simulink library "carnotUIBK"  (R2024b)
settings: Solver=VariableStepAuto  StartTime=0.0  StopTime=10.0  RelTol=1e-3  EnableMultiTasking=on
values from neighbouring files (symbols this model uses):
  area = area + room(kk).area    [THERMALZONE.m]
  boundary = BOUNDARY()    [BUILDING.m]
  building = obj    [BUILDING.m]
  C = zeros(1,length(d)+1)    [CONSTRUCTION.m]
  cp = str2num(value)    [CONSTRUCTION.m]
  pos = find(d_layer>0)    [CONSTRUCTION.m]
  rho = str2num(value)    [CONSTRUCTION.m]
  type = 1    [CONSTRUCTION.m]
  zone = obj.zone(ind)    [THERMALZONE.m]
undefined symbols (not defined in the file or in its folder): A, amb_factor, B, const, control, Dd, get_building, height, p, Qdot_C, Qdot_H, Qdot_I_electricity, Qdot_I_light, Qdot_I_person, Qdot_S, Qdot_T_ground, Qdot_T_neighbour, Qdot_T_opaque, Qdot_T_window, Qdot_V_infiltration, Qdot_V_mech, Qdot_V_window, r_frame, solar_ratio, solar_ratio1, solar_ratio2, Tc, Tr, Ts, Uvalue, view_factor, wall, wallsurface, window, window_height, window_heigth, window_width, windowsurface, x_CO2, x_H2O, x_VOC, z
libraries: carnot x105, $bdroot x22, simulink x18, simulink_extras x14
(part 7 of 13)

== system carnotUIBK/gain/Light/W//light ==
  Switch : Inport
  Constant1 : Constant  Value=zeros(1,13)
  Constant2 : Constant  Value=zeros(1,3)
  Gain1 : Gain  Gain=0.6  SaturateOnIntegerOverflow=on  OutDataTypeStr=Inherit: Same as input  ParamDataTypeStr=Inherit: Same as input
  Gain4 : Gain  Gain=0.4  SaturateOnIntegerOverflow=on  OutDataTypeStr=Inherit: Same as input  ParamDataTypeStr=Inherit: Same as input
  Mux1 : Mux  Inputs=[1 1 13 1 3]
  Product1 : Product
  Profile W/light : carnot/Load/General/Repeating_Profile  period=timevalues(end)  rep_seq_t=timevalues(1:end-1)  rep_seq_d=timeduration  rep_seq_y=values1
      settings: SourceProductName=Carnot
  timeconstant : simulink_extras/Additional Linear/Transfer Fcn (with initial outputs)  N=[1]  D=[60 1]  Y0=0  U0=0
  "[S]" : Outport  VectorParamsAs1DForOutWhenUnconnected=off
  wires:
  Product1/1 -> "[S]"/1
  Switch/1 -> Product1/1
  Gain4/1 -> Mux1/2
  Mux1/1 -> Product1/2
  Gain1/1 -> Mux1/1
  Profile W/light/1 -> timeconstant/1
  Constant1/1 -> Mux1/3
  Constant2/1 -> Mux1/5
  timeconstant/1 -> Mux1/4, Gain4/1, Gain1/1

== system carnotUIBK/gain/Light/W//m² ==
  Switch : Inport
  Constant1 : Constant  Value=zeros(1,13)
  Constant2 : Constant  Value=zeros(1,3)
  Gain1 : Gain  Gain=z.heated_area  SaturateOnIntegerOverflow=on  OutDataTypeStr=Inherit: Same as input  ParamDataTypeStr=Inherit: Same as input
  Gain3 : Gain  Gain=0.6  SaturateOnIntegerOverflow=on  OutDataTypeStr=Inherit: Same as input  ParamDataTypeStr=Inherit: Same as input
  Gain5 : Gain  Gain=0.4  SaturateOnIntegerOverflow=on  OutDataTypeStr=Inherit: Same as input  ParamDataTypeStr=Inherit: Same as input
  Mux2 : Mux  Inputs=[1 1 13 1 3]
  Product : Product
  Profile W/m² : carnot/Load/General/Repeating_Profile  period=timevalues(end)  rep_seq_t=timevalues(1:end-1)  rep_seq_d=timeduration  rep_seq_y=values1
      settings: SourceProductName=Carnot
  timeconstant : simulink_extras/Additional Linear/Transfer Fcn (with initial outputs)  N=[1]  D=[60 1]  Y0=0  U0=0
  "[S]" : Outport  VectorParamsAs1DForOutWhenUnconnected=off
  wires:
  Product/1 -> "[S]"/1
  Switch/1 -> Product/1
  Gain5/1 -> Mux2/2
  Mux2/1 -> Product/2
  Gain3/1 -> Mux2/1
  Profile W/m²/1 -> Gain1/1
  Gain1/1 -> timeconstant/1
  Constant1/1 -> Mux2/3
  Constant2/1 -> Mux2/5
  timeconstant/1 -> Mux2/4, Gain5/1, Gain3/1

== system carnotUIBK/gain/Moisture/kg//s ==
  note: 2500 kJ/kg
  Constant13 : Constant  Value=zeros(1,11)
  Constant14 : Constant  Value=zeros(1,2)
  Constant3 : Constant  Value=zeros(1,2)
  Gain1 : Gain  Gain=1.0  SaturateOnIntegerOverflow=on  OutDataTypeStr=Inherit: Same as input  ParamDataTypeStr=Inherit: Same as input
  Gain2 : Gain  Gain=-2500000  SaturateOnIntegerOverflow=on  OutDataTypeStr=Inherit: Same as input  ParamDataTypeStr=Inherit: Same as input
  Gain4 : Gain  Gain=0.0  SaturateOnIntegerOverflow=on  OutDataTypeStr=Inherit: Same as input  ParamDataTypeStr=Inherit: Same as input
  Mux2 : Mux  Inputs=[1 1 2 1 11 1 2]
  Profile kg/s : carnot/Load/General/Repeating_Profile  period=timevalues(end)  rep_seq_t=timevalues(1:end-1)  rep_seq_d=timeduration  rep_seq_y=values1
      settings: SourceProductName=Carnot
  timeconstant : simulink_extras/Additional Linear/Transfer Fcn (with initial outputs)  N=[1]  D=[60 1]  Y0=0  U0=0
  "[S]" : Outport  VectorParamsAs1DForOutWhenUnconnected=off
  wires:
  Gain4/1 -> Mux2/2
  Mux2/1 -> "[S]"/1
  Gain1/1 -> Mux2/1
  Profile kg/s/1 -> timeconstant/1
  Constant13/1 -> Mux2/5
  Constant14/1 -> Mux2/7
  Constant3/1 -> Mux2/3
  Gain2/1 -> Mux2/6, Gain4/1, Gain1/1
  timeconstant/1 -> Mux2/4, Gain2/1

== system carnotUIBK/gain/People/W//m² ==
  Switch : Inport
  Constant1 : Constant  Value=zeros(1,12)
  Constant2 : Constant  Value=zeros(1,4)
  Gain1 : Gain  Gain=z.heated_area  SaturateOnIntegerOverflow=on  OutDataTypeStr=Inherit: Same as input  ParamDataTypeStr=Inherit: Same as input
  Gain2 : Gain  Gain=0.5  SaturateOnIntegerOverflow=on  OutDataTypeStr=Inherit: Same as input  ParamDataTypeStr=Inherit: Same as input
  Gain4 : Gain  Gain=0.5  SaturateOnIntegerOverflow=on  OutDataTypeStr=Inherit: Same as input  ParamDataTypeStr=Inherit: Same as input
  Mux1 : Mux  Inputs=[1 1 12 1 4]
  Product1 : Product
  profile_1 : carnot/Load/General/Repeating_Profile  period=timevalues(end)  rep_seq_t=timevalues(1:end-1)  rep_seq_d=timeduration  rep_seq_y=values1
      settings: SourceProductName=Carnot
  timeconstant : simulink_extras/Additional Linear/Transfer Fcn (with initial outputs)  N=[1]  D=[60 1]  Y0=0  U0=0
  "[S]" : Outport  VectorParamsAs1DForOutWhenUnconnected=off
  wires:
  Switch/1 -> Product1/1
  Product1/1 -> "[S]"/1
  Gain1/1 -> timeconstant/1
  Gain4/1 -> Mux1/2
  Gain2/1 -> Mux1/1
  Mux1/1 -> Product1/2
  profile_1/1 -> Gain1/1
  Constant1/1 -> Mux1/3
  Constant2/1 -> Mux1/5
  timeconstant/1 -> Gain4/1, Mux1/4, Gain2/1

== system carnotUIBK/gain/People/W//ppl (activity) ==
  Top : Inport
  Switch : Inport  Port=2
  Constant1 : Constant  Value=zeros(1,2)
  Constant2 : Constant  Value=zeros(1,4)
  Constant3 : Constant  Value=zeros(1,8)
  Gain1 : Gain  Gain=0.5  SaturateOnIntegerOverflow=on  OutDataTypeStr=Inherit: Same as input  ParamDataTypeStr=Inherit: Same as input
  Gain2 : Gain  Gain=0.5  SaturateOnIntegerOverflow=on  OutDataTypeStr=Inherit: Same as input  ParamDataTypeStr=Inherit: Same as input
  Gain4 : Gain  Gain=0.5  SaturateOnIntegerOverflow=on  OutDataTypeStr=Inherit: Same as input  ParamDataTypeStr=Inherit: Same as input
  LUT_Qdot_dry : Subsystem
      mask help:
      | This block delivers the SENSITIVE/DRY HEAT POWER one person emitts in a room depending on his activity and the actual sensitive temperature in the middle of a room.
      |
      | Qdot_dry	: sensitive/dry heat power emitted from 1 person, W
      | activity		: number of class of person activity (DIN 1946, VDI 2078):
      | 		   0 - no physical work (sleeping)
      | 		   1 - relaxed work (home, office, school)
      | 		   2 - light physical work, standing (shopping, laboratory)
      | 		   3 - moderately heavy physical activity (home work)
      | 		   4 - heavy physical activity (sports, heavy maschinery)
      | Top		: sensitive/operational temperature in the middle of a
      | 	  	  room/zone,°C
  LUT_Qdot_hum1 : Subsystem  mask(LOOK UP TABLE){}
      mask help:
      | This block delivers the LATENT/HUMID HEAT POWER one person emitts in a room depending on his activity and the actual sensitive temperature in the middle of a room.
      |
      | Qdot_hum	: latent/humid heat power emitted from 1 person, W
      | activity		: number of class of person activity (DIN 1946, VDI 2078):
      | 		   0 - no physical work (sleeping)
      | 		   1 - relaxed work (home, office, school)
      | 		   2 - light physical work standing (shopping, laboratory)
      | 		   3 - moderately heavy physical activity (home work)
      | 		   4 - heavy physical activity (sports, heavy maschinery)
      | Top		: sensitive/operational temperature in the middle of a
      | 		  room/zone,°C
  LUT_mdot_CO2 : Subsystem  mask(LOOK UP TABLE){}
      mask help:
      | This block delivers the CO2 MASS FLOW one person emitts in a room depending on his activity and the actual sensitive temperature in the middle of a room.
      |
      | mdot_CO2	: CO2 mass flow emitted from 1 person, kg/s
      | activity		: number of class of person activity (DIN 1946, VDI 2078):
      | 		   0 - no physical work (sleeping)
      | 		   1 - relaxed work (home, office, school)
      | 		   2 - light physical work standing (shopping, laboratory)
      | 		   3 - moderately heavy physical activity (home work)
      | 		   4 - heavy physical activity (sports, heavy maschinery)
  LUT_mdot_H2O : Subsystem  mask(LOOK UP TABLE){}
      mask help:
      | This block delivers the WATER MASS FLOW one person emitts in a room depending on his activity and the actual sensitive temperature in the middle of a room.
      |
      | mdot_H2O	: water mass flow emitted from 1 person, kg/s
      | activity		: number of class of person activity (DIN 1946, VDI 2078):
      | 		   0 - no physical work (sleeping)
      | 		   1 - relaxed work (home, office, school)
      | 		   2 - light physical work standing (shopping, laboratory)
      | 		   3 - moderately heavy physical activity (home work)
      | 		   4 - heavy physical activity (sports, heavy maschinery)
      | Top		: sensitive/operational temperature in the middle of a
      | 		  room/zone,°C
  Mux1 : Mux  Inputs=[1 1 2 1 1 8 1 4]
  Product{,1..4} (5 alike) : Product
  Sum : Sum  InputSameDT=on  SaturateOnIntegerOverflow=on  OutDataTypeStr=Inherit: Same as first input
  Sum1 : Sum  InputSameDT=on  SaturateOnIntegerOverflow=on  OutDataTypeStr=Inherit: Same as first input
  profile people : carnot/Load/General/Repeating_Profile  period=timevalues(end)  rep_seq_t=timevalues(1:end-1)  rep_seq_d=timeduration  rep_seq_y=values1
      settings: SourceProductName=Carnot
  profile people activity : carnot/Load/General/Repeating_Profile  period=timevalues(end)  rep_seq_t=timevalues(1:end-1)  rep_seq_d=timeduration  rep_seq_y=values2
      settings: SourceProductName=Carnot
  timeconstant{,1..3} (4 alike) : simulink_extras/Additional Linear/Transfer Fcn (with initial outputs)  N=[1]  D=[60 1]  Y0=0  U0=0
  "[S]" : Outport  VectorParamsAs1DForOutWhenUnconnected=off
  wires:
  Top/1 -> LUT_mdot_H2O/2(Top), LUT_Qdot_hum1/2(Top), LUT_Qdot_dry/2(Top)
  Switch/1 -> Product1/1
  Product1/1 -> "[S]"/1
  Sum1/1 -> Mux1/7
  LUT_Qdot_dry/1(Qdot_dry) -> Product2/2
  Product3/1 -> timeconstant1/1  "mdot_H2O"
  Gain4/1 -> Sum/2, Mux1/2  "Qdot_r"
  Product4/1 -> timeconstant/1
  Sum/1 -> Mux1/1  "Qdot_c"
  Mux1/1 -> Product1/2
  LUT_Qdot_hum1/1(Qdot_hum) -> Product/2
  profile people activity/1 -> LUT_mdot_CO2/1(activity), LUT_mdot_H2O/1(activity), LUT_Qdot_dry/1(activity), LUT_Qdot_hum1/1(activity)
  Gain1/1 -> Sum1/1, Sum/1
  Gain2/1 -> Sum1/2, Gain4/1
  profile people/1 -> Product4/1, Product3/1, Product2/1, Product/1
  Product/1 -> timeconstant3/1
  Product2/1 -> timeconstant2/1
  LUT_mdot_CO2/1(mdot_CO2) -> Product4/2
  LUT_mdot_H2O/1(mdot_H2O) -> Product3/2
  Constant1/1 -> Mux1/3
  Constant2/1 -> Mux1/8
  Constant3/1 -> Mux1/6
  timeconstant/1 -> Mux1/5
  timeconstant1/1 -> Mux1/4
  timeconstant2/1 -> Gain2/1
  timeconstant3/1 -> Gain1/1

== system carnotUIBK/gain/People/W//ppl (constant) ==
  Top : Inport
  Switch : Inport  Port=2
  Constant1 : Constant  Value=zeros(1,2)
  Constant2 : Constant  Value=zeros(1,4)
  Constant3 : Constant  Value=zeros(1,8)
  Gain1 : Gain  Gain=10  SaturateOnIntegerOverflow=on  OutDataTypeStr=Inherit: Same as input  ParamDataTypeStr=Inherit: Same as input
  Gain2 : Gain  Gain=50  SaturateOnIntegerOverflow=on  OutDataTypeStr=Inherit: Same as input  ParamDataTypeStr=Inherit: Same as input
  Gain4 : Gain  Gain=0.5  SaturateOnIntegerOverflow=on  OutDataTypeStr=Inherit: Same as input  ParamDataTypeStr=Inherit: Same as input
  LUT_mdot_CO2 : Subsystem  mask(LOOK UP TABLE){}
      mask help:
      | This block delivers the CO2 MASS FLOW one person emitts in a room depending on his activity and the actual sensitive temperature in the middle of a room.
      |
      | mdot_CO2	: CO2 mass flow emitted from 1 person, kg/s
      | activity		: number of class of person activity (DIN 1946, VDI 2078):
      | 		   0 - no physical work (sleeping)
      | 		   1 - relaxed work (home, office, school)
      | 		   2 - light physical work standing (shopping, laboratory)
      | 		   3 - moderately heavy physical activity (home work)
      | 		   4 - heavy physical activity (sports, heavy maschinery)
  LUT_mdot_H2O : Subsystem  mask(LOOK UP TABLE){}
      mask help:
      | This block delivers the WATER MASS FLOW one person emitts in a room depending on his activity and the actual sensitive temperature in the middle of a room.
      |
      | mdot_H2O	: water mass flow emitted from 1 person, kg/s
      | activity		: number of class of person activity (DIN 1946, VDI 2078):
      | 		   0 - no physical work (sleeping)
      | 		   1 - relaxed work (home, office, school)
      | 		   2 - light physical work standing (shopping, laboratory)
      | 		   3 - moderately heavy physical activity (home work)
      | 		   4 - heavy physical activity (sports, heavy maschinery)
      | Top		: sensitive/operational temperature in the middle of a
      | 		  room/zone,°C
  Mux1 : Mux  Inputs=[1 1 2 1 1 8 1 4]
  Product1 : Product
  Product3 : Product
  Product4 : Product
  Sum : Sum  InputSameDT=on  SaturateOnIntegerOverflow=on  OutDataTypeStr=Inherit: Same as first input
  Sum1 : Sum  InputSameDT=on  SaturateOnIntegerOverflow=on  OutDataTypeStr=Inherit: Same as first input
  profile people : carnot/Load/General/Repeating_Profile  period=timevalues(end)  rep_seq_t=timevalues(1:end-1)  rep_seq_d=timeduration  rep_seq_y=values1
      settings: SourceProductName=Carnot
  profile people activity : carnot/Load/General/Repeating_Profile  period=timevalues(end)  rep_seq_t=timevalues(1:end-1)  rep_seq_d=timeduration  rep_seq_y=values2
      settings: SourceProductName=Carnot
  timeconstant{,1..3} (4 alike) : simulink_extras/Additional Linear/Transfer Fcn (with initial outputs)  N=[1]  D=[60 1]  Y0=0  U0=0
  "[S]" : Outport  VectorParamsAs1DForOutWhenUnconnected=off
  wires:
  Product1/1 -> "[S]"/1
  Switch/1 -> Product1/1
  Top/1 -> LUT_mdot_H2O/2(Top)
  Sum1/1 -> Mux1/7
  profile people/1 -> Product4/1, Product3/1, Gain2/1, Gain1/1
  Product3/1 -> timeconstant/1  "mdot_H2O"
  Gain4/1 -> Mux1/2, Sum/2  "Qdot_r"
  Product4/1 -> timeconstant1/1
  Sum/1 -> Mux1/1  "Qdot_c"
  Mux1/1 -> Product1/2
  Gain1/1 -> timeconstant3/1
  Gain2/1 -> timeconstant2/1
  profile people activity/1 -> LUT_mdot_CO2/1(activity), LUT_mdot_H2O/1(activity)
  Constant1/1 -> Mux1/3
  Constant2/1 -> Mux1/8
  Constant3/1 -> Mux1/6
  LUT_mdot_H2O/1(mdot_H2O) -> Product3/2  "mdot_H2O"
  LUT_mdot_CO2/1(mdot_CO2) -> Product4/2
  timeconstant/1 -> Mux1/4
  timeconstant1/1 -> Mux1/5
  timeconstant2/1 -> Gain4/1, Sum1/2
  timeconstant3/1 -> Sum/1, Sum1/1

== system carnotUIBK/infiltration/infiltration_constant/Subsystem ==
  note: ASSUMPTION: mdot_air_out2in = mdot_air_in2out !
  note: (kg/kg)
  note: (kg/kg)
  note: (kg/s)
  note: (kg/s)
  note: (kg/s)
  mdot_air : Inport
  x_in : Inport  Port=2
  x_out : Inport  Port=3
  Demux2 : Demux  Outputs=2
      settings: DisplayOption=none
  Demux3 : Demux  Outputs=2
      settings: DisplayOption=none
  Fcn{,1..3} (4 alike) : Fcn  Expr=u / (1+u)
  Product5 : Product  InputSameDT=on  SaturateOnIntegerOverflow=on  OutDataTypeStr=Inherit: Same as first input
  Product6 : Product  InputSameDT=on  SaturateOnIntegerOverflow=on  OutDataTypeStr=Inherit: Same as first input
  Sum1 : Sum  Inputs=+-  InputSameDT=on  SaturateOnIntegerOverflow=on  OutDataTypeStr=Inherit: Same as first input
  Sum2 : Sum  Inputs=+-  InputSameDT=on  SaturateOnIntegerOverflow=on  OutDataTypeStr=Inherit: Same as first input
  mdot_H2O : Outport  InitialOutput=0  VectorParamsAs1DForOutWhenUnconnected=off
  mdot_CO2 : Outport  Port=2  InitialOutput=0  VectorParamsAs1DForOutWhenUnconnected=off
  wires:
  Product5/1 -> mdot_H2O/1
  Product6/1 -> mdot_CO2/1
  mdot_air/1 -> Product5/1, Product6/1  "mdot_air >=0"
  Sum1/1 -> Product5/2
  Sum2/1 -> Product6/2
  Fcn3/1 -> Sum2/2
  Fcn1/1 -> Sum2/1
  Fcn2/1 -> Sum1/2
  Fcn/1 -> Sum1/1
  x_in/1 -> Demux3/1
  Demux3/1 -> Fcn2/1  "x_H2O_in"
  Demux3/2 -> Fcn3/1  "x_CO2_in"
  Demux2/2 -> Fcn1/1  "x_CO2_out"
  Demux2/1 -> Fcn/1  "x_H2O_out"
  x_out/1 -> Demux2/1

== system carnotUIBK/infiltration/infiltration_constant/Window_Ventilation ==
  Troom : Inport
  Tamb : Inport  Port=2
  control : Inport  Port=3
  Mux : Mux  Inputs=3
  S-Function : S-Function  FunctionName=tiltvent  Parameters=alpha, H, W  SFunctionDeploymentMode=off  EnableBusSupport=off
  V_rate [m^3/s] : Outport  VectorParamsAs1DForOutWhenUnconnected=off
  wires:
  Troom/1 -> Mux/1
  Mux/1 -> S-Function/1
  S-Function/1 -> V_rate [m^3/s]/1
  control/1 -> Mux/3
  Tamb/1 -> Mux/2

== system carnotUIBK/infiltration/infiltration_pressure/infiltration_pressure ==
  T_room : Inport
  WDB : Inport  Port=2
  H_window : Inport  Port=3
  facade_angle : Inport  Port=4
  add_coeff_wind : Inport  Port=5
  Add : Sum
  Bus Selector : BusSelector  OutputSignals=Temperature_Ambient,Station_Pressure,Wind_Speed,Wind_Direction
  Divide : Product  Inputs=*//
  Divide1 : Product  Inputs=**/
  K : Constant  Value=273.15
  Ra : Constant  Value=287.058
  dP_infiltration : Subsystem
  delta_p : Constant  Value=50
  n : Constant  Value=0.66
  n50 : Constant  Value=n50
  pow_law : Math  Operator=pow  SignedPower=on
  power_law_infiltration : Subsystem
  volume : Constant  Value=volume
  m_dot : Outport  VectorParamsAs1DForOutWhenUnconnected=off
  wires:
  power_law_infiltration/1(m_dot) -> m_dot/1
  dP_infiltration/1(dP_total) -> power_law_infiltration/1(dP)
  T_room/1 -> dP_infiltration/1(T_int)
  WDB/1 -> Bus Selector/1
  Bus Selector/1 -> Add/1, dP_infiltration/2(T_ext)  "<Temperature_Ambient>"
  Bus Selector/3 -> dP_infiltration/3(windspeed)  "<Wind_Speed>"
  Bus Selector/4 -> dP_infiltration/4(wind_angle)  "<Wind_Direction>"
  Bus Selector/2 -> Divide/1  "<Station_Pressure>"
  H_window/1 -> dP_infiltration/6(H_window)
  Ra/1 -> Divide/2
  K/1 -> Add/2
  Add/1 -> Divide/3
  n/1 -> power_law_infiltration/3(n), pow_law/2
  Divide/1 -> power_law_infiltration/4(density), dP_infiltration/5(air_density_ext)
  facade_angle/1 -> dP_infiltration/8(facade_angle)
  add_coeff_wind/1 -> dP_infiltration/7(add_coeff_wind)
  Divide1/1 -> power_law_infiltration/2(C)
  n50/1 -> Divide1/1
  pow_law/1 -> Divide1/3
  delta_p/1 -> pow_law/1
  volume/1 -> Divide1/2

== system carnotUIBK/room_node/1-node/mass blalance ==
  mdot_H2O : Inport
  mdot_CO2 : Inport  Port=2
  mdot_VOC : Inport  Port=3
  AIB : Inport  Port=4
  (1/m^3) : Constant  Value=1/zoneairvolume
  Bus Selector1 : BusSelector  OutputSignals=rho
  m_CO2 : Integrator  InitialCondition=zonestartCO2  LimitOutput=on  LowerSaturationLimit=0
  m_H2O : Integrator  InitialCondition=zonestartWATER  LimitOutput=on  LowerSaturationLimit=0
  m_VOC : Integrator  InitialCondition=zonestartVOC  LimitOutput=on  LowerSaturationLimit=0
  x1 : Product  Inputs=**  InputSameDT=on  SaturateOnIntegerOverflow=on  OutDataTypeStr=Inherit: Same as first input
  x2 : Product  Inputs=**  InputSameDT=on  SaturateOnIntegerOverflow=on  OutDataTypeStr=Inherit: Same as first input
  x3 : Product  Inputs=**  InputSameDT=on  SaturateOnIntegerOverflow=on  OutDataTypeStr=Inherit: Same as first input
  x4 : Product  Inputs=*/  InputSameDT=on  SaturateOnIntegerOverflow=on  OutDataTypeStr=Inherit: Same as first input
  x_H2O : Outport  VectorParamsAs1DForOutWhenUnconnected=off
  x_CO2 : Outport  Port=2  VectorParamsAs1DForOutWhenUnconnected=off
  x_VOC : Outport  Port=3  VectorParamsAs1DForOutWhenUnconnected=off
  wires:
  Bus Selector1/1 -> x4/2  "<rho>"
  AIB/1 -> Bus Selector1/1
  mdot_VOC/1 -> m_VOC/1
  m_CO2/1 -> x2/1
  m_VOC/1 -> x3/1
  x4/1 -> x3/2, x2/2, x1/2
  m_H2O/1 -> x1/1
  x3/1 -> x_VOC/1  "x_VOC"
  (1/m^3)/1 -> x4/1
  x2/1 -> x_CO2/1  "x_CO2"
  x1/1 -> x_H2O/1  "x_H2O"
  mdot_H2O/1 -> m_H2O/1
  mdot_CO2/1 -> m_CO2/1

== system carnotUIBK/room_node/1-node/pressure ==
  mdot_air : Inport
  AIB : Inport  Port=2
  (1/m^3) : Constant  Value=1/zoneairvolume
  Bus Selector1 : BusSelector  OutputSignals=Tc
  Subsystem : Subsystem
  Transfer Fcn (with initial outputs)1 : Subsystem  mask(Transfer Function with Initial Outputs){N=[1], D=[timeconst  1], Y0=zonestartP0, U0=1}
      mask prompts: N "Numerator:"; D "Denominator:"; Y0 "Initial output:"; U0 "Initial input:"
      mask help: Vector expressions for numerator, and denominator. Coefficients are in descending powers of s.
      mask init:
      | [A,B,C,Dd]=tf2ss(N,D);if (isempty(Y0));[m,n]=size(A);X0=zeros(1,m); end; if (isempty(U0));[m,p]=size(B);U0=zeros(1,p);end;X0=getxo(A,B,C,Dd,U0,Y0,0);
      mask Help: Specify the initial output for the transfer function.  An optimization routine attempts to determine the appropriate initial states so that the specified initial output is achieved.  For more details, see the m-file getxo.m
      mask Display: dpoly(N,D,'s')
  m_air : Integrator  InitialCondition=zonestartAIR  LimitOutput=on  LowerSaturationLimit=0
  x : Product  Inputs=***  InputSameDT=on  SaturateOnIntegerOverflow=on  OutDataTypeStr=Inherit: Same as first input
  p : Outport  VectorParamsAs1DForOutWhenUnconnected=off
  wires:
  Transfer Fcn (with initial outputs)1/1(Out1) -> p/1  "p"
  Subsystem/1(R*T ') -> x/2
  (1/m^3)/1 -> x/3
  m_air/1 -> x/1
  AIB/1 -> Bus Selector1/1
  Bus Selector1/1 -> Subsystem/1(T)  "<Tc>"
  x/1 -> Transfer Fcn (with initial outputs)1/1(In1)
  mdot_air/1 -> m_air/1

== system carnotUIBK/room_node/1-node/sensitive_node ==
  note: SENSITIVE node
  Qdotc : Inport
  Qdotr : Inport  Port=2
  Add : Sum
  Integrator : Integrator  InitialCondition=zonestartTEMP
  mcp : Constant  Value=1/mcp
  x3 : Product  Inputs=**  InputSameDT=on  SaturateOnIntegerOverflow=on  OutDataTypeStr=Inherit: Same as first input
  Tc : Outport  VectorParamsAs1DForOutWhenUnconnected=off
  wires:
  x3/1 -> Integrator/1
  Integrator/1 -> Tc/1
  Add/1 -> x3/1
  Qdotc/1 -> Add/2
  Qdotr/1 -> Add/1
  mcp/1 -> x3/2

== system carnotUIBK/room_node/1-node_womass/sensitive_node ==
  note: SENSITIVE node
  Qdotc : Inport
  Qdotr : Inport  Port=2
  Add : Sum
  Integrator : Integrator  InitialCondition=zonestartTEMP
  mcp : Constant  Value=1/mcp
  x3 : Product  Inputs=**  InputSameDT=on  SaturateOnIntegerOverflow=on  OutDataTypeStr=Inherit: Same as first input
  Tc : Outport  VectorParamsAs1DForOutWhenUnconnected=off
  wires:
  x3/1 -> Integrator/1
  Integrator/1 -> Tc/1
  Add/1 -> x3/1
  Qdotc/1 -> Add/2
  Qdotr/1 -> Add/1
  mcp/1 -> x3/2

== system carnotUIBK/room_node/2-node/Sensitive room temperature ==
  note: Sensitive temperature
  Tr : Inport
  Tc : Inport  Port=2
  1-share_c : Gain  Gain=1-share_c  SaturateOnIntegerOverflow=on  OutDataTypeStr=Inherit: Same as input  ParamDataTypeStr=Inherit: Same as input
  Sum : Sum  InputSameDT=on  SaturateOnIntegerOverflow=on  OutDataTypeStr=Inherit: Same as first input
  share_c : Gain  Gain=share_c  SaturateOnIntegerOverflow=on  OutDataTypeStr=Inherit: Same as input  ParamDataTypeStr=Inherit: Same as input
  Ts : Outport  VectorParamsAs1DForOutWhenUnconnected=off
  wires:
  Tr/1 -> 1-share_c/1
  Tc/1 -> share_c/1
  share_c/1 -> Sum/1  "Tc"
  1-share_c/1 -> Sum/2  "Tr"
  Sum/1 -> Ts/1

== system carnotUIBK/room_node/2-node/convective_node ==
  note: CONVECTIVE node
  Qdotc : Inport
  AIB : Inport  Port=2
  (1/m^3) : Constant  Value=1/zoneairvolume
  Bus Selector1 : BusSelector  OutputSignals=rho,cp
  Integrator : Integrator  InitialCondition=zonestartTEMP
  x3 : Product  Inputs=**  InputSameDT=on  SaturateOnIntegerOverflow=on  OutDataTypeStr=Inherit: Same as first input
  x4 : Product  Inputs=*//  InputSameDT=on  SaturateOnIntegerOverflow=on  OutDataTypeStr=Inherit: Same as first input
  Tc : Outport  VectorParamsAs1DForOutWhenUnconnected=off
  wires:
  Bus Selector1/2 -> x4/3  "<cp>"
  Bus Selector1/1 -> x4/2  "<rho>"
  AIB/1 -> Bus Selector1/1
  x3/1 -> Integrator/1
  (1/m^3)/1 -> x4/1
  x4/1 -> x3/2
  Integrator/1 -> Tc/1
  Qdotc/1 -> x3/1

== system carnotUIBK/room_node/2-node/density and capacity ==
  T : Inport
  p : Inport  Port=2
  fluid_type : Inport  Port=3
  fluid_mix : Inport  Port=4
  Add : Sum  Inputs=2
  Constant1 : Constant  Value=10000
  Constant2 : Constant  Value=0.0001
  Divide : Product  Inputs=*/
  K : Constant  Value=273.15
  Product : Product
  Product1 : Product
  Ra : Gain  Gain=287.058
  Rounding Function : Rounding
  Terminator : Terminator
  Terminator1 : Terminator
  Transfer Fcn (with initial outputs) : Subsystem  mask(Transfer Function with Initial Outputs){N=[1], D=[timeconst  1], Y0=1.1893, U0=1}
      mask prompts: N "Numerator:"; D "Denominator:"; Y0 "Initial output:"; U0 "Initial input:"
      mask help: Vector expressions for numerator, and denominator. Coefficients are in descending powers of s.
      mask init:
      | [A,B,C,Dd]=tf2ss(N,D);if (isempty(Y0));[m,n]=size(A);X0=zeros(1,m); end; if (isempty(U0));[m,p]=size(B);U0=zeros(1,p);end;X0=getxo(A,B,C,Dd,U0,Y0,0);
      mask Help: Specify the initial output for the transfer function.  An optimization routine attempts to determine the appropriate initial states so that the specified initial output is achieved.  For more details, see the m-file getxo.m
      mask Display: dpoly(N,D,'s')
  cp_const : Constant  Value=1006.8
  rho : Outport  VectorParamsAs1DForOutWhenUnconnected=off
  cp : Outport  Port=2  VectorParamsAs1DForOutWhenUnconnected=off
  wires:
  cp_const/1 -> cp/1
  Divide/1 -> Transfer Fcn (with initial outputs)/1(In1)
  p/1 -> Divide/1
  fluid_type/1 -> Terminator/1
  fluid_mix/1 -> Terminator1/1
  T/1 -> Add/1
  K/1 -> Add/2
  Add/1 -> Ra/1
  Ra/1 -> Divide/2
  Rounding Function/1 -> Product1/1
  Transfer Fcn (with initial outputs)/1(Out1) -> Product/1
  Product/1 -> Rounding Function/1
  Constant1/1 -> Product/2
  Constant2/1 -> Product1/2
  Product1/1 -> rho/1

== system carnotUIBK/room_node/2-node/mass blalance ==
  mdot_H2O : Inport
  mdot_CO2 : Inport  Port=2
  mdot_VOC : Inport  Port=3
  AIB : Inport  Port=4
  (1/m^3) : Constant  Value=1/zoneairvolume
  Bus Selector1 : BusSelector  OutputSignals=rho
  m_CO2 : Integrator  InitialCondition=zonestartCO2  LimitOutput=on  LowerSaturationLimit=0
  m_H2O : Integrator  InitialCondition=zonestartWATER  LimitOutput=on  LowerSaturationLimit=0
  m_VOC : Integrator  InitialCondition=zonestartVOC  LimitOutput=on  LowerSaturationLimit=0
  x1 : Product  Inputs=**  InputSameDT=on  SaturateOnIntegerOverflow=on  OutDataTypeStr=Inherit: Same as first input
  x2 : Product  Inputs=**  InputSameDT=on  SaturateOnIntegerOverflow=on  OutDataTypeStr=Inherit: Same as first input
  x3 : Product  Inputs=**  InputSameDT=on  SaturateOnIntegerOverflow=on  OutDataTypeStr=Inherit: Same as first input
  x4 : Product  Inputs=*/  InputSameDT=on  SaturateOnIntegerOverflow=on  OutDataTypeStr=Inherit: Same as first input
  x_H2O : Outport  VectorParamsAs1DForOutWhenUnconnected=off
  x_CO2 : Outport  Port=2  VectorParamsAs1DForOutWhenUnconnected=off
  x_VOC : Outport  Port=3  VectorParamsAs1DForOutWhenUnconnected=off
  wires:
  Bus Selector1/1 -> x4/2  "<rho>"
  AIB/1 -> Bus Selector1/1
  mdot_VOC/1 -> m_VOC/1
  m_CO2/1 -> x2/1
  m_VOC/1 -> x3/1
  x4/1 -> x3/2, x2/2, x1/2
  m_H2O/1 -> x1/1
  x3/1 -> x_VOC/1  "x_VOC"
  (1/m^3)/1 -> x4/1
  x2/1 -> x_CO2/1  "x_CO2"
  x1/1 -> x_H2O/1  "x_H2O"
  mdot_H2O/1 -> m_H2O/1
  mdot_CO2/1 -> m_CO2/1

== system carnotUIBK/room_node/2-node/pressure ==
  mdot_air : Inport
  AIB : Inport  Port=2
  (1/m^3) : Constant  Commented=on  Value=1/zoneairvolume
  Bus Selector1 : BusSelector  Commented=on  OutputSignals=Tc
  Subsystem : Subsystem  Commented=on
  Transfer Fcn (with initial outputs)1 : Subsystem  Commented=on  mask(Transfer Function with Initial Outputs){N=[1], D=[timeconst  1], Y0=zonestartP0, U0=1}
      mask prompts: N "Numerator:"; D "Denominator:"; Y0 "Initial output:"; U0 "Initial input:"
      mask help: Vector expressions for numerator, and denominator. Coefficients are in descending powers of s.
      mask init:
      | [A,B,C,Dd]=tf2ss(N,D);if (isempty(Y0));[m,n]=size(A);X0=zeros(1,m); end; if (isempty(U0));[m,p]=size(B);U0=zeros(1,p);end;X0=getxo(A,B,C,Dd,U0,Y0,0);
      mask Help: Specify the initial output for the transfer function.  An optimization routine attempts to determine the appropriate initial states so that the specified initial output is achieved.  For more details, see the m-file getxo.m
      mask Display: dpoly(N,D,'s')
  convert2U32 : DataTypeConversion  Commented=on  OutDataTypeStr=uint32  SaturateOnIntegerOverflow=off  RndMeth=Floor
  convert2double : DataTypeConversion  Commented=on  OutDataTypeStr=double  SaturateOnIntegerOverflow=off  RndMeth=Floor
  m_air : Integrator  Commented=on  InitialCondition=zonestartAIR  LimitOutput=on  LowerSaturationLimit=0
  p0 : Constant  Value=1e5
  x : Product  Commented=on  Inputs=***  InputSameDT=on  SaturateOnIntegerOverflow=on  OutDataTypeStr=Inherit: Same as first input
  p : Outport  VectorParamsAs1DForOutWhenUnconnected=off
  wires:
  Transfer Fcn (with initial outputs)1/1(Out1) -> convert2U32/1  "p"
  Subsystem/1(R*T ') -> x/2
  (1/m^3)/1 -> x/3
  m_air/1 -> x/1
  AIB/1 -> Bus Selector1/1
  Bus Selector1/1 -> Subsystem/1(T)  "<Tc>"
  x/1 -> Transfer Fcn (with initial outputs)1/1(In1)
  mdot_air/1 -> m_air/1
  convert2U32/1 -> convert2double/1
  p0/1 -> p/1

== system carnotUIBK/room_node/2-node/radiative_node ==
  note: RADIATIVE node
  Qdotr : Inport
  Gain : Gain  Gain=1/timeconst
  Integrator : Integrator  InitialCondition=zonestartTEMP
  Tr : Outport  VectorParamsAs1DForOutWhenUnconnected=off
  wires:
  Integrator/1 -> Tr/1
  Qdotr/1 -> Gain/1
  Gain/1 -> Integrator/1

== system carnotUIBK/room_node/2-node_ideal/Sensitive room temperature ==
  note: Sensitive temperature
  Tr : Inport
  Tc : Inport  Port=2
  1-share_c : Gain  Gain=1-share_c  SaturateOnIntegerOverflow=on  OutDataTypeStr=Inherit: Same as input  ParamDataTypeStr=Inherit: Same as input
  Sum : Sum  InputSameDT=on  SaturateOnIntegerOverflow=on  OutDataTypeStr=Inherit: Same as first input
  share_c : Gain  Gain=share_c  SaturateOnIntegerOverflow=on  OutDataTypeStr=Inherit: Same as input  ParamDataTypeStr=Inherit: Same as input
  Ts : Outport  VectorParamsAs1DForOutWhenUnconnected=off
  wires:
  Tr/1 -> 1-share_c/1
  Tc/1 -> share_c/1
  share_c/1 -> Sum/1  "Tc"
  1-share_c/1 -> Sum/2  "Tr"
  Sum/1 -> Ts/1

== system carnotUIBK/room_node/2-node_ideal/mass blalance ==
  mdot_H2O : Inport
  mdot_CO2 : Inport  Port=2
  mdot_VOC : Inport  Port=3
  AIB : Inport  Port=4
  (1/m^3) : Constant  Value=1/zoneairvolume
  Bus Selector1 : BusSelector  OutputSignals=rho
  m_CO2 : Integrator  InitialCondition=zonestartCO2  LimitOutput=on  LowerSaturationLimit=0
  m_H2O : Integrator  InitialCondition=zonestartWATER  LimitOutput=on  LowerSaturationLimit=0
  m_VOC : Integrator  InitialCondition=zonestartVOC  LimitOutput=on  LowerSaturationLimit=0
  x1 : Product  Inputs=**  InputSameDT=on  SaturateOnIntegerOverflow=on  OutDataTypeStr=Inherit: Same as first input
  x2 : Product  Inputs=**  InputSameDT=on  SaturateOnIntegerOverflow=on  OutDataTypeStr=Inherit: Same as first input
  x3 : Product  Inputs=**  InputSameDT=on  SaturateOnIntegerOverflow=on  OutDataTypeStr=Inherit: Same as first input
  x4 : Product  Inputs=*/  InputSameDT=on  SaturateOnIntegerOverflow=on  OutDataTypeStr=Inherit: Same as first input
  x_H2O : Outport  VectorParamsAs1DForOutWhenUnconnected=off
  x_CO2 : Outport  Port=2  VectorParamsAs1DForOutWhenUnconnected=off
  x_VOC : Outport  Port=3  VectorParamsAs1DForOutWhenUnconnected=off
  wires:
  Bus Selector1/1 -> x4/2  "<rho>"
  AIB/1 -> Bus Selector1/1
  mdot_VOC/1 -> m_VOC/1
  m_CO2/1 -> x2/1
  m_VOC/1 -> x3/1
  x4/1 -> x3/2, x2/2, x1/2
  m_H2O/1 -> x1/1
  x3/1 -> x_VOC/1  "x_VOC"
  (1/m^3)/1 -> x4/1
  x2/1 -> x_CO2/1  "x_CO2"
  x1/1 -> x_H2O/1  "x_H2O"
  mdot_H2O/1 -> m_H2O/1
  mdot_CO2/1 -> m_CO2/1

== system carnotUIBK/room_node/2-node_ideal/pressure ==
  mdot_air : Inport
  AIB : Inport  Port=2
  (1/m^3) : Constant  Value=1/zoneairvolume
  Bus Selector1 : BusSelector  OutputSignals=Tc
  Subsystem : Subsystem
  Transfer Fcn (with initial outputs)1 : Subsystem  mask(Transfer Function with Initial Outputs){N=[1], D=[timeconst  1], Y0=zonestartP0, U0=1}
      mask prompts: N "Numerator:"; D "Denominator:"; Y0 "Initial output:"; U0 "Initial input:"
      mask help: Vector expressions for numerator, and denominator. Coefficients are in descending powers of s.
      mask init:
      | [A,B,C,Dd]=tf2ss(N,D);if (isempty(Y0));[m,n]=size(A);X0=zeros(1,m); end; if (isempty(U0));[m,p]=size(B);U0=zeros(1,p);end;X0=getxo(A,B,C,Dd,U0,Y0,0);
      mask Help: Specify the initial output for the transfer function.  An optimization routine attempts to determine the appropriate initial states so that the specified initial output is achieved.  For more details, see the m-file getxo.m
      mask Display: dpoly(N,D,'s')
  m_air : Integrator  InitialCondition=zonestartAIR  LimitOutput=on  LowerSaturationLimit=0
  x : Product  Inputs=***  InputSameDT=on  SaturateOnIntegerOverflow=on  OutDataTypeStr=Inherit: Same as first input
  p : Outport  VectorParamsAs1DForOutWhenUnconnected=off
  wires:
  Transfer Fcn (with initial outputs)1/1(Out1) -> p/1  "p"
  Subsystem/1(R*T ') -> x/2
  (1/m^3)/1 -> x/3
  m_air/1 -> x/1
  AIB/1 -> Bus Selector1/1
  Bus Selector1/1 -> Subsystem/1(T)  "<Tc>"
  x/1 -> Transfer Fcn (with initial outputs)1/1(In1)
  mdot_air/1 -> m_air/1

== system carnotUIBK/room_node/EMPTY/AIB_initialize ==
  Bus Creator2 : BusCreator  Inputs=9
  Constant{,1..8} (9 alike) : Constant  Value=0
  AIB : Outport  VectorParamsAs1DForOutWhenUnconnected=off
  wires:
  Bus Creator2/1 -> AIB/1
  Constant4/1 -> Bus Creator2/5  "x_CO2"
  Constant2/1 -> Bus Creator2/3  "Tr"
  Constant1/1 -> Bus Creator2/2  "Tc"
  Constant6/1 -> Bus Creator2/7  "rho"
  Constant7/1 -> Bus Creator2/8  "cp"
  Constant/1 -> Bus Creator2/1  "Ts"
  Constant8/1 -> Bus Creator2/9  "p"
  Constant3/1 -> Bus Creator2/4  "x_H2O"
  Constant5/1 -> Bus Creator2/6  "x_VOC"

== system carnotUIBK/room_node/EMPTY/BDB_initialize ==
  Bus Creator2 : BusCreator  Inputs=13
  Constant{,1..12} (13 alike) : Constant  Value=0
  BDB : Outport  VectorParamsAs1DForOutWhenUnconnected=off
  wires:
  Constant2/1 -> Bus Creator2/3  "Qdot_T_neighbour"
  Constant9/1 -> Bus Creator2/10  "Qdot_I_light"
  Constant4/1 -> Bus Creator2/5  "Qdot_V_mech"
  Constant1/1 -> Bus Creator2/2  "Qdot_T_ground"
  Constant3/1 -> Bus Creator2/4  "Qdot_T_window"
  Constant10/1 -> Bus Creator2/11  "Qdot_I_electricity"
  Constant12/1 -> Bus Creator2/13  "Qdot_C"
  Constant11/1 -> Bus Creator2/12  "Qdot_H"
  Constant7/1 -> Bus Creator2/9  "Qdot_I_person"
  Constant6/1 -> Bus Creator2/7  "Qdot_V_infiltration"
  Constant/1 -> Bus Creator2/1  "Qdot_T_opaque"
  Constant8/1 -> Bus Creator2/8  "Qdot_S"
  Constant5/1 -> Bus Creator2/6  "Qdot_V_window"
  Bus Creator2/1 -> BDB/1

== system carnotUIBK/room_node/EMPTY/Sensitive room temperature ==
  note: Sensitive temperature
  Tr : Inport
  Tc : Inport  Port=2
  1-share_c : Gain  Gain=1-share_c  SaturateOnIntegerOverflow=on  OutDataTypeStr=Inherit: Same as input  ParamDataTypeStr=Inherit: Same as input
  Sum : Sum  InputSameDT=on  SaturateOnIntegerOverflow=on  OutDataTypeStr=Inherit: Same as first input
  share_c : Gain  Gain=share_c  SaturateOnIntegerOverflow=on  OutDataTypeStr=Inherit: Same as input  ParamDataTypeStr=Inherit: Same as input
  Ts : Outport  VectorParamsAs1DForOutWhenUnconnected=off
  wires:
  Tr/1 -> 1-share_c/1
  Tc/1 -> share_c/1
  share_c/1 -> Sum/1  "Tc"
  1-share_c/1 -> Sum/2  "Tr"
  Sum/1 -> Ts/1

== system carnotUIBK/wall_intersection/R-C model/alpha_i1 ==
  Ts : Inport
  AIB : Inport  Port=2
  Qdot sol : Inport  Port=3
  phis : Inport  Port=4
  alpha_i_down : Subsystem  VariantControl=V_i_XXX_XXX_wXXX_hti2  mask(ALFA){}
      mask help:
      | Convective and radiative heat transfer at the INDOOR SURFACE of a VERTICAL OUTER WALL.
      |
      | [AIV] : conditions of zone node,
      | Ts : temperature of wall surface, °C,
      | qdots : specific heat flow into wall construction, W/m^2,
      | [S] : heat and air flow to zone node.
  alpha_i_horizontal : Subsystem  VariantControl=V_i_XXX_XXX_wXXX_hti0  mask(ALFA){}
      mask help:
      | Convective and radiative heat transfer at the INDOOR SURFACE of a VERTICAL OUTER WALL.
      |
      | [AIV] : conditions of zone node,
      | Ts : temperature of wall surface, °C,
      | qdots : specific heat flow into wall construction, W/m^2,
      | [S] : heat and air flow to zone node.
  alpha_i_up : Subsystem  VariantControl=V_i_XXX_XXX_wXXX_hti1  mask(ALFA){}
      mask help:
      | Convective and radiative heat transfer at the INDOOR SURFACE of a VERTICAL OUTER WALL.
      |
      | [AIV] : conditions of zone node,
      | Ts : temperature of wall surface, °C,
      | qdots : specific heat flow into wall construction, W/m^2,
      | [S] : heat and air flow to zone node.
  qdots : Outport  VectorParamsAs1DForOutWhenUnconnected=off
  "[S]" : Outport  Port=2  VectorParamsAs1DForOutWhenUnconnected=off
  alpha_c : Outport  Port=3  VectorParamsAs1DForOutWhenUnconnected=off
  phi_i_1/100 : Outport  Port=4  VectorParamsAs1DForOutWhenUnconnected=off

== system carnotUIBK/wall_intersection/R-C model/alpha_i2 ==
  Ts : Inport
  AIB : Inport  Port=2
  Qdot sol : Inport  Port=3
  phis : Inport  Port=4
  alpha_i_down : Subsystem  VariantControl=V_i_XXX_XXX_wXXX_hti2  mask(ALFA){}
      mask help:
      | Convective and radiative heat transfer at the INDOOR SURFACE of a VERTICAL OUTER WALL.
      |
      | [AIV] : conditions of zone node,
      | Ts : temperature of wall surface, °C,
      | qdots : specific heat flow into wall construction, W/m^2,
      | [S] : heat and air flow to zone node.
  alpha_i_horizontal : Subsystem  VariantControl=V_i_XXX_XXX_wXXX_hti0  mask(ALFA){}
      mask help:
      | Convective and radiative heat transfer at the INDOOR SURFACE of a VERTICAL OUTER WALL.
      |
      | [AIV] : conditions of zone node,
      | Ts : temperature of wall surface, °C,
      | qdots : specific heat flow into wall construction, W/m^2,
      | [S] : heat and air flow to zone node.
  alpha_i_up : Subsystem  VariantControl=V_i_XXX_XXX_wXXX_hti1  mask(ALFA){}
      mask help:
      | Convective and radiative heat transfer at the INDOOR SURFACE of a VERTICAL OUTER WALL.
      |
      | [AIV] : conditions of zone node,
      | Ts : temperature of wall surface, °C,
      | qdots : specific heat flow into wall construction, W/m^2,
      | [S] : heat and air flow to zone node.
  qdots : Outport  VectorParamsAs1DForOutWhenUnconnected=off
  "[S]" : Outport  Port=2  VectorParamsAs1DForOutWhenUnconnected=off
  alpha_c : Outport  Port=3  VectorParamsAs1DForOutWhenUnconnected=off
  phi_i_1/100 : Outport  Port=4  VectorParamsAs1DForOutWhenUnconnected=off

== system carnotUIBK/wall_intersection/UA/Rsi ==
  down : Subsystem  VariantControl=V_i_XXX_XXX_wXXX_hti2
  horizontal : Subsystem  VariantControl=V_i_XXX_XXX_wXXX_hti0
  up : Subsystem  VariantControl=V_i_XXX_XXX_wXXX_hti1
  Rsi : Outport  VectorParamsAs1DForOutWhenUnconnected=off

== system carnotUIBK/wall_intersection/hygrothermal model/alpha_i1 ==
  Ts : Inport
  AIB : Inport  Port=2
  Qdot sol : Inport  Port=3
  phis : Inport  Port=4
  alpha_i_down : Subsystem  VariantControl=V_i_XXX_XXX_wXXX_hti2  mask(ALFA){}
      mask help:
      | Convective and radiative heat transfer at the INDOOR SURFACE of a VERTICAL OUTER WALL.
      |
      | [AIV] : conditions of zone node,
      | Ts : temperature of wall surface, °C,
      | qdots : specific heat flow into wall construction, W/m^2,
      | [S] : heat and air flow to zone node.
  alpha_i_horizontal : Subsystem  VariantControl=V_i_XXX_XXX_wXXX_hti0  mask(ALFA){}
      mask help:
      | Convective and radiative heat transfer at the INDOOR SURFACE of a VERTICAL OUTER WALL.
      |
      | [AIV] : conditions of zone node,
      | Ts : temperature of wall surface, °C,
      | qdots : specific heat flow into wall construction, W/m^2,
      | [S] : heat and air flow to zone node.
  alpha_i_up : Subsystem  VariantControl=V_i_XXX_XXX_wXXX_hti1  mask(ALFA){}
      mask help:
      | Convective and radiative heat transfer at the INDOOR SURFACE of a VERTICAL OUTER WALL.
      |
      | [AIV] : conditions of zone node,
      | Ts : temperature of wall surface, °C,
      | qdots : specific heat flow into wall construction, W/m^2,
      | [S] : heat and air flow to zone node.
  qdots : Outport  VectorParamsAs1DForOutWhenUnconnected=off
  "[S]" : Outport  Port=2  VectorParamsAs1DForOutWhenUnconnected=off
  alpha_c : Outport  Port=3  VectorParamsAs1DForOutWhenUnconnected=off
  phi_i_1/100 : Outport  Port=4  VectorParamsAs1DForOutWhenUnconnected=off

== system carnotUIBK/wall_intersection/hygrothermal model/alpha_i2 ==
  Ts : Inport
  AIB : Inport  Port=2
  Qdot sol : Inport  Port=3
  phis : Inport  Port=4
  alpha_i_down : Subsystem  VariantControl=V_i_XXX_XXX_wXXX_hti2  mask(ALFA){}
      mask help:
      | Convective and radiative heat transfer at the INDOOR SURFACE of a VERTICAL OUTER WALL.
      |
      | [AIV] : conditions of zone node,
      | Ts : temperature of wall surface, °C,
      | qdots : specific heat flow into wall construction, W/m^2,
      | [S] : heat and air flow to zone node.
  alpha_i_horizontal : Subsystem  VariantControl=V_i_XXX_XXX_wXXX_hti0  mask(ALFA){}
      mask help:
      | Convective and radiative heat transfer at the INDOOR SURFACE of a VERTICAL OUTER WALL.
      |
      | [AIV] : conditions of zone node,
      | Ts : temperature of wall surface, °C,
      | qdots : specific heat flow into wall construction, W/m^2,
      | [S] : heat and air flow to zone node.
  alpha_i_up : Subsystem  VariantControl=V_i_XXX_XXX_wXXX_hti1  mask(ALFA){}
      mask help:
      | Convective and radiative heat transfer at the INDOOR SURFACE of a VERTICAL OUTER WALL.
      |
      | [AIV] : conditions of zone node,
      | Ts : temperature of wall surface, °C,
      | qdots : specific heat flow into wall construction, W/m^2,
      | [S] : heat and air flow to zone node.
  qdots : Outport  VectorParamsAs1DForOutWhenUnconnected=off
  "[S]" : Outport  Port=2  VectorParamsAs1DForOutWhenUnconnected=off
  alpha_c : Outport  Port=3  VectorParamsAs1DForOutWhenUnconnected=off
  phi_i_1/100 : Outport  Port=4  VectorParamsAs1DForOutWhenUnconnected=off

== system carnotUIBK/wall_zone/R-C model/alpha_e ==
  WDB : Inport
  GDB : Inport  Port=2
  NDB : Inport  Port=3
  AIB : Inport  Port=4
  Ts : Inport  Port=5
  Qdot_sol : Inport  Port=6
  phis : Inport  Port=7
  alpha_e_AMBIENT : Subsystem  VariantControl=V_zXXX_wXXX_hte0  mask(ALFA){}
      mask help:
      | Convective and radiative HEAT TRANSFER at the WEATHER EXPOSED SURFACE of an OUTER WALL.
      |
      | [W*] : modified weather data, adapted to height over ground,
      | Ts : temperature of outdoor wall surface, °C,
      | qdots : specific heat flow into wall / window construction, W/m^2.
  alpha_e_GROUND : Subsystem  VariantControl=V_zXXX_wXXX_hte1  mask(ALFA){}
      mask help:
      | Convective and radiative HEAT TRANSFER at the WEATHER EXPOSED SURFACE of an OUTER WALL.
      |
      | [W*] : modified weather data, adapted to height over ground,
      | Ts : temperature of outdoor wall surface, °C,
      | qdots : specific heat flow into wall / window construction, W/m^2.
  alpha_e_INTERNAL : Subsystem  VariantControl=V_zXXX_wXXX_hte2  mask(ALFA){}
      mask help:
      | Convective and radiative HEAT TRANSFER at the WEATHER EXPOSED SURFACE of an OUTER WALL.
      |
      | [W*] : modified weather data, adapted to height over ground,
      | Ts : temperature of outdoor wall surface, °C,
      | qdots : specific heat flow into wall / window construction, W/m^2.
  alpha_e_NEIGHBOUR : Subsystem  VariantControl=V_zXXX_wXXX_hte3  mask(ALFA){}
      mask help:
      | Convective and radiative HEAT TRANSFER at the WEATHER EXPOSED SURFACE of an OUTER WALL.
      |
      | [W*] : modified weather data, adapted to height over ground,
      | Ts : temperature of outdoor wall surface, °C,
      | qdots : specific heat flow into wall / window construction, W/m^2.
  qdots : Outport  VectorParamsAs1DForOutWhenUnconnected=off
  "[S]" : Outport  Port=2  VectorParamsAs1DForOutWhenUnconnected=off
  alpha_c : Outport  Port=3  VectorParamsAs1DForOutWhenUnconnected=off
  phi_e_1/100 : Outport  Port=4  VectorParamsAs1DForOutWhenUnconnected=off
  theta_e : Outport  Port=5  VectorParamsAs1DForOutWhenUnconnected=off

== system carnotUIBK/wall_zone/R-C model/alpha_i ==
  Ts : Inport
  AIB : Inport  Port=2
  Qdot sol : Inport  Port=3
  phis : Inport  Port=4
  alpha_i_down : Subsystem  VariantControl=V_zXXX_wXXX_hti2  mask(ALFA){}
      mask help:
      | Convective and radiative heat transfer at the INDOOR SURFACE of a VERTICAL OUTER WALL.
      |
      | [AIV] : conditions of zone node,
      | Ts : temperature of wall surface, °C,
      | qdots : specific heat flow into wall construction, W/m^2,
      | [S] : heat and air flow to zone node.
  alpha_i_horizontal : Subsystem  VariantControl=V_zXXX_wXXX_hti0  mask(ALFA){}
      mask help:
      | Convective and radiative heat transfer at the INDOOR SURFACE of a VERTICAL OUTER WALL.
      |
      | [AIV] : conditions of zone node,
      | Ts : temperature of wall surface, °C,
      | qdots : specific heat flow into wall construction, W/m^2,
      | [S] : heat and air flow to zone node.
  alpha_i_up : Subsystem  VariantControl=V_zXXX_wXXX_hti1  mask(ALFA){}
      mask help:
      | Convective and radiative heat transfer at the INDOOR SURFACE of a VERTICAL OUTER WALL.
      |
      | [AIV] : conditions of zone node,
      | Ts : temperature of wall surface, °C,
      | qdots : specific heat flow into wall construction, W/m^2,
      | [S] : heat and air flow to zone node.
  qdots : Outport  VectorParamsAs1DForOutWhenUnconnected=off
  "[S]" : Outport  Port=2  VectorParamsAs1DForOutWhenUnconnected=off
  alpha_c : Outport  Port=3  VectorParamsAs1DForOutWhenUnconnected=off
  phi_i_1/100 : Outport  Port=4  VectorParamsAs1DForOutWhenUnconnected=off

== system carnotUIBK/wall_zone/UA/Rse ==
  WDB : Inport
  GDB : Inport  Port=2
  NDB : Inport  Port=3
  AIB : Inport  Port=4
  Qdot_sol : Inport  Port=5
  Qdot_in : Inport  Port=6
  R : Inport  Port=7
  Rsi : Inport  Port=8
  AMBIENT : Subsystem  VariantControl=V_zXXX_wXXX_hte0
  GROUND : Subsystem  VariantControl=V_zXXX_wXXX_hte1
  INTERNAL : Subsystem  VariantControl=V_zXXX_wXXX_hte2
  NEIGHBOUR : Subsystem  VariantControl=V_zXXX_wXXX_hte3
  "[S]" : Outport  VectorParamsAs1DForOutWhenUnconnected=off

== system carnotUIBK/wall_zone/UA/Rsi ==
  down : Subsystem  VariantControl=V_zXXX_wXXX_hti2
  horizontal : Subsystem  VariantControl=V_zXXX_wXXX_hti0
  up : Subsystem  VariantControl=V_zXXX_wXXX_hti1
  Rsi : Outport  VectorParamsAs1DForOutWhenUnconnected=off

== system carnotUIBK/wall_zone/hygrothermal model/alpha_e ==
  WDB : Inport
  GDB : Inport  Port=2
  NDB : Inport  Port=3
  AIB : Inport  Port=4
  Ts : Inport  Port=5
  Qdot_sol : Inport  Port=6
  phis : Inport  Port=7
  alpha_e_AMBIENT : Subsystem  VariantControl=V_zXXX_wXXX_hte0  mask(ALFA){}
      mask help:
      | Convective and radiative HEAT TRANSFER at the WEATHER EXPOSED SURFACE of an OUTER WALL.
      |
      | [W*] : modified weather data, adapted to height over ground,
      | Ts : temperature of outdoor wall surface, °C,
      | qdots : specific heat flow into wall / window construction, W/m^2.
  alpha_e_GROUND : Subsystem  VariantControl=V_zXXX_wXXX_hte1  mask(ALFA){}
      mask help:
      | Convective and radiative HEAT TRANSFER at the WEATHER EXPOSED SURFACE of an OUTER WALL.
      |
      | [W*] : modified weather data, adapted to height over ground,
      | Ts : temperature of outdoor wall surface, °C,
      | qdots : specific heat flow into wall / window construction, W/m^2.
  alpha_e_INTERNAL : Subsystem  VariantControl=V_zXXX_wXXX_hte2  mask(ALFA){}
      mask help:
      | Convective and radiative HEAT TRANSFER at the WEATHER EXPOSED SURFACE of an OUTER WALL.
      |
      | [W*] : modified weather data, adapted to height over ground,
      | Ts : temperature of outdoor wall surface, °C,
      | qdots : specific heat flow into wall / window construction, W/m^2.
  alpha_e_NEIGHBOUR : Subsystem  VariantControl=V_zXXX_wXXX_hte3  mask(ALFA){}
      mask help:
      | Convective and radiative HEAT TRANSFER at the WEATHER EXPOSED SURFACE of an OUTER WALL.
      |
      | [W*] : modified weather data, adapted to height over ground,
      | Ts : temperature of outdoor wall surface, °C,
      | qdots : specific heat flow into wall / window construction, W/m^2.
  qdots : Outport  VectorParamsAs1DForOutWhenUnconnected=off
  "[S]" : Outport  Port=2  VectorParamsAs1DForOutWhenUnconnected=off
  alpha_c : Outport  Port=3  VectorParamsAs1DForOutWhenUnconnected=off
  phi_e_1/100 : Outport  Port=4  VectorParamsAs1DForOutWhenUnconnected=off
  theta_e : Outport  Port=5  VectorParamsAs1DForOutWhenUnconnected=off

== system carnotUIBK/wall_zone/hygrothermal model/alpha_i ==
  Ts : Inport
  AIB : Inport  Port=2
  Qdot sol : Inport  Port=3
  phis : Inport  Port=4
  alpha_i_down : Subsystem  VariantControl=V_zXXX_wXXX_hti2  mask(ALFA){}
      mask help:
      | Convective and radiative heat transfer at the INDOOR SURFACE of a VERTICAL OUTER WALL.
      |
      | [AIV] : conditions of zone node,
      | Ts : temperature of wall surface, °C,
      | qdots : specific heat flow into wall construction, W/m^2,
      | [S] : heat and air flow to zone node.
  alpha_i_horizontal : Subsystem  VariantControl=V_zXXX_wXXX_hti0  mask(ALFA){}
      mask help:
      | Convective and radiative heat transfer at the INDOOR SURFACE of a VERTICAL OUTER WALL.
      |
      | [AIV] : conditions of zone node,
      | Ts : temperature of wall surface, °C,
      | qdots : specific heat flow into wall construction, W/m^2,
      | [S] : heat and air flow to zone node.
  alpha_i_up : Subsystem  VariantControl=V_zXXX_wXXX_hti1  mask(ALFA){}
      mask help:
      | Convective and radiative heat transfer at the INDOOR SURFACE of a VERTICAL OUTER WALL.
      |
      | [AIV] : conditions of zone node,
      | Ts : temperature of wall surface, °C,
      | qdots : specific heat flow into wall construction, W/m^2,
      | [S] : heat and air flow to zone node.
  qdots : Outport  VectorParamsAs1DForOutWhenUnconnected=off
  "[S]" : Outport  Port=2  VectorParamsAs1DForOutWhenUnconnected=off
  alpha_c : Outport  Port=3  VectorParamsAs1DForOutWhenUnconnected=off
  phi_i_1/100 : Outport  Port=4  VectorParamsAs1DForOutWhenUnconnected=off
